simulink model "ECE385_Project_Final"  (R2024a)
settings: Solver=VariableStepAuto  StartTime=0.0  StopTime=1  RelTol=1e-3
model workspace (MAT data in the model file):
  R = 10000
libraries: spsCurrentMeasurementLib x1, spsDCMachineLib x1, spsDCVoltageSourceLib x1, spsGroundLib x1, spsAsynchronousMachineSIUnitsLib x1, spsPowerLib x1, spsSeriesRLCBranchLib x1, spsThreePhaseProgrammableVoltageSourceLib x1, spsVoltageMeasurementLib x1, sps_lib x1
settings Model: Creator=SIU856538288  LastModifiedBy=noahb
settings SolverCC: AlgebraicLoopSolver=TrustRegion
settings DebuggingCC: ArithmeticOperatorsInVariantConditions=warning
settings ModelReferenceCC: EnableRefExpFcnMdlSchedulingChecks=on
settings SFSimCC: CustomCodeUndefinedFunction=UseInterfaceOnly
settings RTWCC: GPUComputeCapability=3.5

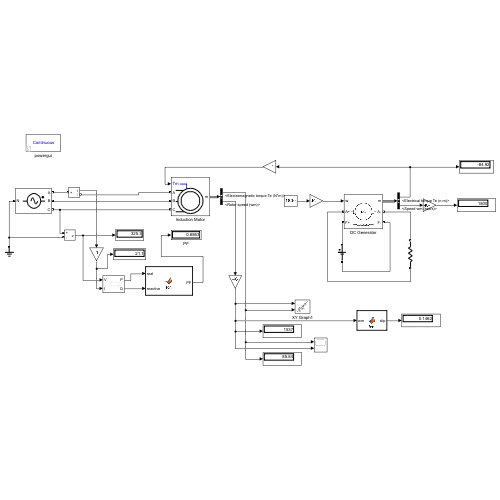
[thumbnail: Simulink's stored preview of the top-level diagram]
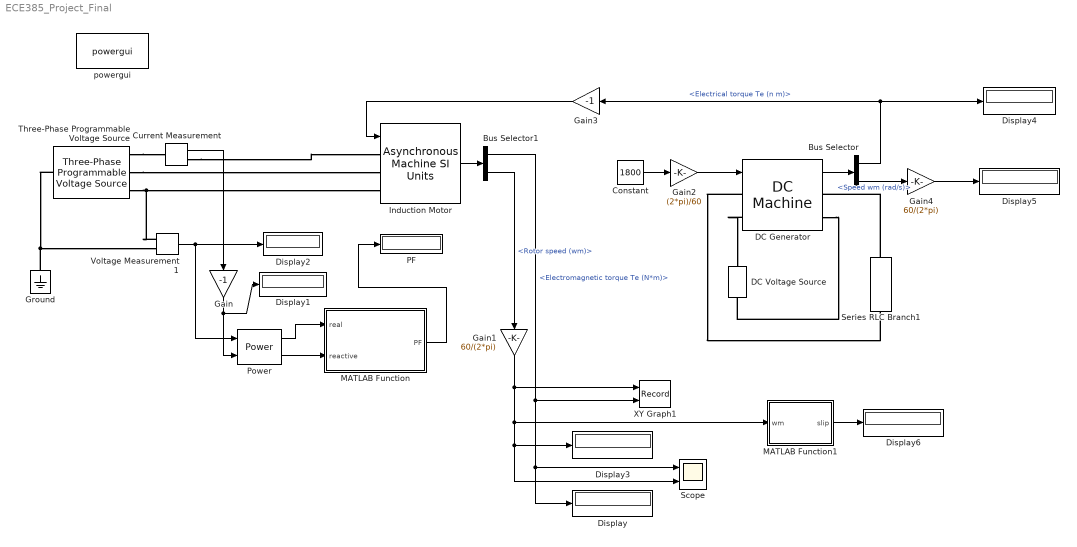
== system ECE385_Project_Final ==
  Bus Selector : BusSelector  OutputSignals=Electrical torque Te (n m),Speed wm (rad/s)
  Bus Selector1 : BusSelector  OutputSignals=Mechanical.Electromagnetic torque Te (N*m),Mechanical.Rotor speed (wm)
  Constant : Constant  Value=1800
  Current Measurement : spsCurrentMeasurementLib/Current Measurement  PhasorSimulation=off  OutputType=Complex  PSBequivalent=0
  DC Generator : spsDCMachineLib/DC Machine  PresetModel=No  MechanicalLoad=Speed w  FieldType=Wound  ShowDetailedParameters=on  MeasurementBus=off  RLa=[0.78 0.016]  RLf=[150 112.5]  Laf=1.234  MachineConstant=Torque constant (N.m/A)  Ke=1.8  Kt=1.8  J=0.05  Bm=0.01  Tf=0  w0=1  Ifinit=1  TsPowergui=0  TsBlock=-1
  DC Voltage Source : spsDCVoltageSourceLib/DC Voltage Source  Amplitude=150  Measurements=None
  Display{,1..6} (7 alike) : Display
  Gain : Gain  Gain=-1
  Gain1 : Gain  Gain=60/(2*pi)
  Gain2 : Gain  Gain=(2*pi)/60
  Gain3 : Gain  Gain=-1
  Gain4 : Gain  Gain=60/(2*pi)
  Ground : spsGroundLib/Ground  LConnTagsString=a
  Induction Motor : spsAsynchronousMachineSIUnitsLib/Asynchronous Machine SI Units  RotorType=Squirrel-cage  PresetModel="01:  5 HP   460 V 60Hz 1750 RPM"  MechanicalLoad=Torque Tm  ShowDetailedParameters=on  ReferenceFrame=Rotor  Units=SI  MeasurementBus=off  NominalParameters=[3730 460 60]  VoltageRatio=1  Stator=[1.115 0.005974]  Rotor=[1.083 0.005974]  Cage1=[0.4155 0.002066]  Cage2=[0.4168 0.0003495]  Lm=0.2037  Mechanical=[0.02 0.005752 2]  PolePairs=2  InitialConditions=[0 0 0 0 0 0 0 0]  SimulateSaturation=off  Saturation=[14.03593122, 27.81365428, 53.79336849, 72.68890987, 97.98006896, 148.6815601, 215.7428561, 302.9841135, 428.7778367 ; 230, 322, 414, 460, 506, 552, 598, 644, 690]  LoadFlowParameters=1492000  TsPowergui=0  TsBlock=-1  IterativeModel=Trapezoidal non iterative  IterativeDiscreteModel=Trapezoidal non iterative  Pmec=1.492e+006
  MATLAB Function : MATLAB Function  TreatAsAtomicUnit=on
  MATLAB Function1 : MATLAB Function  TreatAsAtomicUnit=on
  PF : Display
  Power : spsPowerLib/Power  Freq=60  Vinit=[0, 0]  Iinit=[0, 0]  Ts=0
  Scope : Scope  NumInputPorts=2
  Series RLC Branch1 : spsSeriesRLCBranchLib/Series RLC Branch  LConnTagsString=__new0  RConnTagsString=__new0  BranchType=R  Resistance=2.6  Inductance=100  SetiL0=off  InitialCurrent=0  Capacitance=25e-6  Setx0=off  InitialVoltage=0  Measurements=None
  Three-Phase Programmable Voltage Source : spsThreePhaseProgrammableVoltageSourceLib/Three-Phase Programmable Voltage Source  PositiveSequence="[460  0 60]"  VariationEntity=None  VariationType=Table of time-amplitude pairs  VariationTypeAlt=Step  VariationStep=0.5  VariationRate=10  VariationMagnitude=0.3  VariationFrequency=2  VariationTiming=[1 2]  VariationPhaseA=off  Amplitudes=[1 0.8 1.2 1.0]  TimeValues=[0 0.1 0.15 0.2]  HarmonicGeneration=off  HarmonicA=[3 0.2 -25 0]  HarmonicB=[2 0.15 35 2]  Timing="[0.05  3]"  BusType=swing  Pref=0  Qref=0  Qmin=-inf  Qmax=inf
  Voltage Measurement1 : spsVoltageMeasurementLib/Voltage Measurement  PhasorSimulation=off  OutputType=Complex  PSBequivalent=0
  XY Graph1 : Record  FileSettingsInternal="{\"entries\":[{\"content\":{\"excelSettings\":{\"content\":{},\"type\":\"Streamout.ExcelSettings\"}},\"type\":\"Streamout.FileSettingStorage\",\"uuid\":\"\"}],\"packageUris\":[\"http:\\/\\/schema.mathworks.com\\/mf0\\/streamout_blocks\\/R2020a\"],\"version\":\"1.0\"}"  Layout=[1 1]  SignalsInternal="{\"entries\":[{\"content\":{\"signals\":[{\"content\":{\"blockPath\":[],\"dimensions\":[1],\"domain\":\"\",\"lineColor\":\"#a2142f\",\"plots\":[ 1 ],\"port\":1,\"sid\":[\"\"],\"signalID\":1,\"signalName\":\"Gain1\"},\"type\":\"RecordBlkView.Signal\",\"uuid\":\"\"},{\"content\":{\"blockPath\":[],\"dimensions\":[1],\"domain\":\"\",\"lineColor\":\"#139fff\",\"plots\":[ 1 ],\"port\":2,\"sid\":[\"\"],\"signalID\":2,\"signalName\":\"<Electromagnetic torque Te (N*m)>\"},\"type\":\"RecordBlkView.Signal\",\"uuid\":\"\"}]},\"type\":\"RecordBlkView.InputSignals\",\"uuid\":\"\"}],\"packageUris\":[\"http:\\/\\/schema.mathworks.com\\/mf0\\/streamout_blocks\\/R2020a\"],\"version\":\"1.0\"}"  VisualizationBindings="{\"xyplotplugin\":{\"info\":[{\"series\":[{\"bindingParametersList\":[{\"parameter\":\"X-Axis\",\"signalID\":1,\"signalName\":\"Gain1\"},{\"parameter\":\"Y-Axis\",\"signalID\":2,\"signalName\":\"<Electromagnetic torque Te (N*m)>\"}],\"seriesID\":0}],\"subplotID\":1}]}}"  CompatibilityTag=XY
  powergui : sps_lib/powergui  Priority=1  SimulationMode=Continuous  SampleTime=50e-6  frequency=60  Iterations=50  frequencyindice=60  Pbase=100e6  ErrMax=1e-4  UnitsV=kV  UnitsW=MW  buscounter=0  FunctionMessages=off  echomessages=off  EnableUseOfTLC=off  CurrentSourceSwitches=off  DisableSnubberDevices=off  DisableRonSwitches=off  DisableVfSwitches=off  DisplayEquations=off  AutomaticDiscreteSolvers=off  SolverType=Tustin/Backward Euler (TBE)  Interpol=off  ExternalGateDelay=off  methode=off  Ts=100  x0status=blocks  SPID=on  SwTol=0  HookPort=off  NonlinearTolerance=1e-4  nMaxIteration=100  ContinueOnMaxIteration=off  RestoreLinks=warning  ResistiveCurrentMeasurement=off  Frange=[0:2:500]  Ylog=off  Xlog=on  ShowGrid=off  save=off  variable=ZData  structure=0  ZoomFFT=off  StartTime=0.0  cycles=1  DisplayStyle=1  fundamental=60  FreqAxis=off  MaxFrequency=1000  frequencyindicesteady=1  RmsSteady=1  display=off
  wires:
  Bus Selector1/2 -> Gain1/1  "<Rotor speed (wm)>"
  Induction Motor/1 -> Bus Selector1/1
  Bus Selector1/1 -> XY Graph1/2, Display/1, Scope/1  "<Electromagnetic torque Te (N*m)>"
  Gain1/1 -> Scope/2, Display3/1, MATLAB Function1/1(wm), XY Graph1/1
  DC Generator/1 -> Bus Selector/1
  Voltage Measurement1/1 -> Power/1, Display2/1
  Power/2 -> MATLAB Function/2(reactive)
  Current Measurement/1 -> Gain/1
  Power/1 -> MATLAB Function/1(real)
  Gain/1 -> Power/2, Display1/1
  Bus Selector/1 -> Display4/1, Gain3/1  "<Electrical torque Te (n m)>"
  Bus Selector/2 -> Gain4/1  "<Speed wm (rad/s)>"
  Gain4/1 -> Display5/1
  Gain3/1 -> Induction Motor/1
  Constant/1 -> Gain2/1
  MATLAB Function1/1(slip) -> Display6/1
  Gain2/1 -> DC Generator/1
  MATLAB Function/1(PF) -> PF/1
  connections:
  DC Generator/LConn2 -- DC Voltage Source/RConn1
  DC Generator/RConn2 -- DC Voltage Source/LConn1
  Series RLC Branch1/LConn1 -- DC Generator/RConn1
  DC Generator/LConn1 -- Series RLC Branch1/RConn1
  Three-Phase Programmable Voltage Source/RConn3 -- Voltage Measurement1/LConn1 -- Induction Motor/LConn3
  Three-Phase Programmable Voltage Source/RConn1 -- Current Measurement/LConn1
  Current Measurement/RConn1 -- Induction Motor/LConn1
  Three-Phase Programmable Voltage Source/LConn1 -- Ground/LConn1 -- Voltage Measurement1/LConn2
  Three-Phase Programmable Voltage Source/RConn2 -- Induction Motor/LConn2

== matlab function ECE385_Project_Final/MATLAB Function ==
  data: real input; PF output; reactive input
function PF = fcn(real, reactive)

S = sqrt((real^2)+(reactive^2));

PF = real/S;

== matlab function ECE385_Project_Final/MATLAB Function1 ==
  data: wm input; slip output
function slip = fcn(wm)

slip = (1800-wm)/1800;
